simulink model "Acc_Dec_Detection"  (R2021b)
settings: Solver=FixedStepAuto  StartTime=0.0  StopTime=10.0  FixedStep=1  RelTol=1e-3
libraries: simulink x4
settings Model: Creator=HP  LastModifiedBy=HP

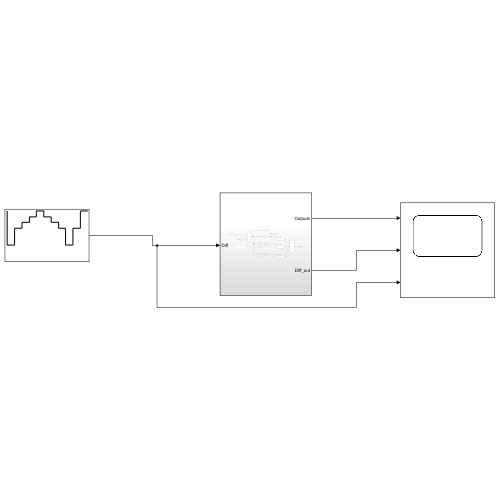
[thumbnail: Simulink's stored preview of the top-level diagram]
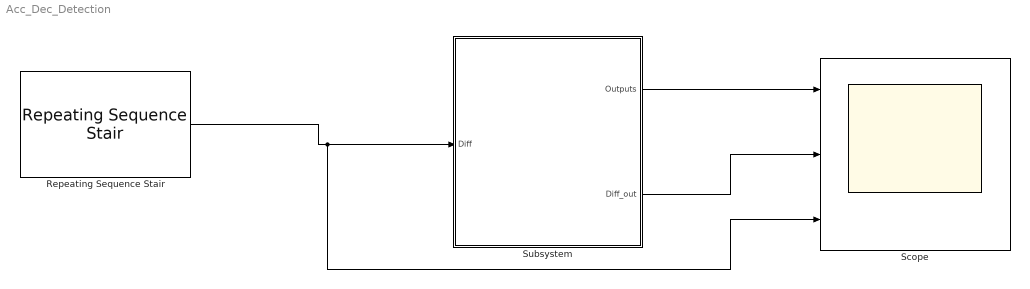
== system Acc_Dec_Detection ==
  Repeating Sequence Stair : simulink/Sources/Repeating Sequence Stair  OutValues=[60 61.5 62 62.5 63 62.5 62 61.5 60 61.5 63 ].'  tsamp=-1  OutMin=[]  OutMax=[]  OutDataTypeStr=double  OutputDataTypeScalingMode=double  OutDataType=fixdt(0,8)  ConRadixGroup=Best Precision: Vector-wise  OutScaling=2^-12
  Scope : Scope  NumInputPorts=3
  Subsystem : Subsystem
  wires:
  Repeating Sequence Stair/1 -> Scope/3, Subsystem/1(Diff)
  Subsystem/1(Outputs) -> Scope/1
  Subsystem/2(Diff_out) -> Scope/2

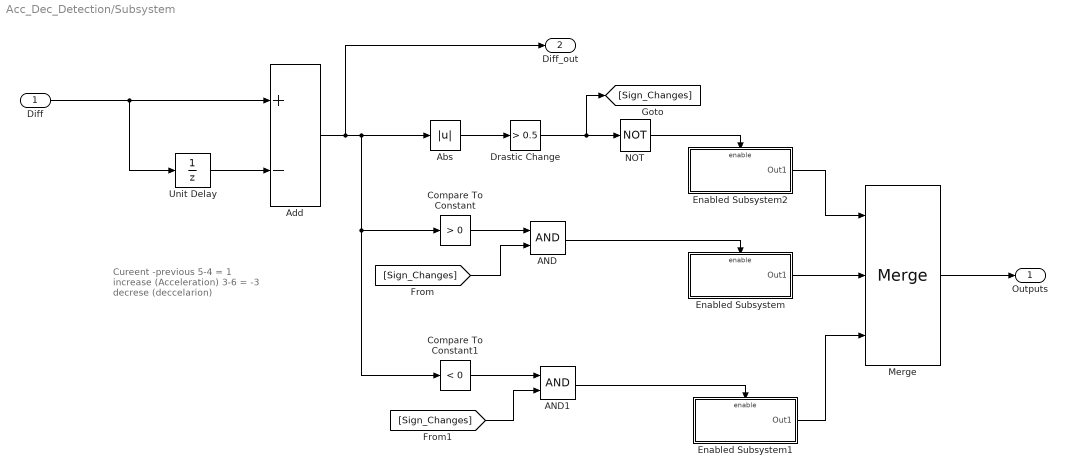
== system Acc_Dec_Detection/Subsystem ==
  note: Cureent -previous
      | 5-4 = 1 increase (Acceleration)
      | 3-6 = -3 decrese (deccelarion)
  Diff : Inport
  AND : Logic  AllPortsSameDT=off  OutDataTypeStr=boolean
  AND1 : Logic  AllPortsSameDT=off  OutDataTypeStr=boolean
  Abs : Abs
  Add : Sum  Inputs=+-
  Compare To Constant : simulink/Logic and Bit Operations/Compare To Constant  relop=>  const=0  OutDataTypeStr=boolean
  Compare To Constant1 : simulink/Logic and Bit Operations/Compare To Constant  relop=<  const=0  OutDataTypeStr=boolean
  Drastic Change : simulink/Logic and Bit Operations/Compare To Constant  relop=>  const=0.5  OutDataTypeStr=boolean
  Enabled Subsystem : Subsystem  TreatAsAtomicUnit=on
  Enabled Subsystem1 : Subsystem  TreatAsAtomicUnit=on
  Enabled Subsystem2 : Subsystem  TreatAsAtomicUnit=on
  Merge : Merge  Inputs=3
  NOT : Logic  Operator=NOT  AllPortsSameDT=off  OutDataTypeStr=boolean
  Unit Delay : UnitDelay  InitialCondition=60  SampleTime=-1  HasFrameUpgradeWarning=on
  Outputs : Outport
  Diff_out : Outport  Port=2
  wires:
  Abs/1 -> Drastic Change/1
  Compare To Constant1/1 -> AND1/1
  Diff/1 -> Unit Delay/1, Add/1
  Enabled Subsystem2/1(Out1) -> Merge/1
  Drastic Change/1 -> [Sign_Changes], NOT/1
  Unit Delay/1 -> Add/2
  AND1/1 -> Enabled Subsystem1/Enable
  Add/1 -> Diff_out/1, Abs/1, Compare To Constant1/1, Compare To Constant/1
  Enabled Subsystem/1(Out1) -> Merge/2
  Compare To Constant/1 -> AND/1
  [Sign_Changes] -> AND/2
  AND/1 -> Enabled Subsystem/Enable
  Merge/1 -> Outputs/1
  Enabled Subsystem1/1(Out1) -> Merge/3
  [Sign_Changes] -> AND1/2
  NOT/1 -> Enabled Subsystem2/Enable

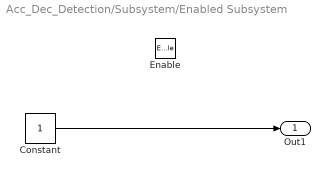
== system Acc_Dec_Detection/Subsystem/Enabled Subsystem ==
  Enable : EnablePort
  Constant : Constant
  Out1 : Outport
  wires:
  Constant/1 -> Out1/1

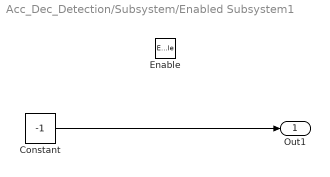
== system Acc_Dec_Detection/Subsystem/Enabled Subsystem1 ==
  Enable : EnablePort
  Constant : Constant  Value=-1
  Out1 : Outport
  wires:
  Constant/1 -> Out1/1

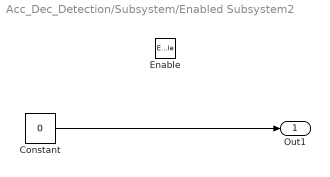
== system Acc_Dec_Detection/Subsystem/Enabled Subsystem2 ==
  Enable : EnablePort
  Constant : Constant  Value=0
  Out1 : Outport
  wires:
  Constant/1 -> Out1/1
